simulink model "Modele_Lineaire_Asservi"  (R2024a)
settings: Solver=VariableStepAuto  StartTime=0.0  StopTime=10  RelTol=1e-3
values from neighbouring files (symbols this model uses):
  den_bille_simu = [5*L_plaque 0]    [Code.m]    (also in Initialisation.m = [7*L_plaque 0])
  den_mot_simu = [R_m*J_eq  (R_m*B_eq+n_g*n_m*k_m*k_t*K_g.^2)]    [Code.m]    (also in Initialisation.m)
  Fig_in = 0    [Code.m]
  Frequence = pi    (= 3.14159265359)    [Code.m]
  K_int = real((((-1)*den_mot(1)*(Inter^2)) + ((-1)*den_mot(2)*(Inter^1))) / (num_mot(1)))    [Code.m]    (also in Initialisation.m)
  num_bille_simu = [3*g*r_arm]    [Code.m]    (also in Initialisation.m = [5*g*r_arm])
  num_mot_simu = [K_g*n_m*n_g*k_t]    [Code.m]    (also in Initialisation.m)
  Test_Position = 0.06    [Code.m]    (also in Initialisation.m)
  X_den = TF_PD_Bode_Den    [Code.m]    (also in Initialisation.m)
  X_num = TF_PD_Bode_Num    [Code.m]    (also in Initialisation.m)
settings Model: Creator=francoisdesautels  LastModifiedBy=francoisdesautels

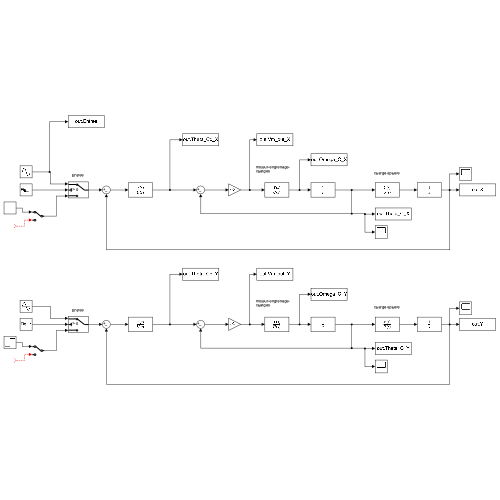
[thumbnail: Simulink's stored preview of the top-level diagram]
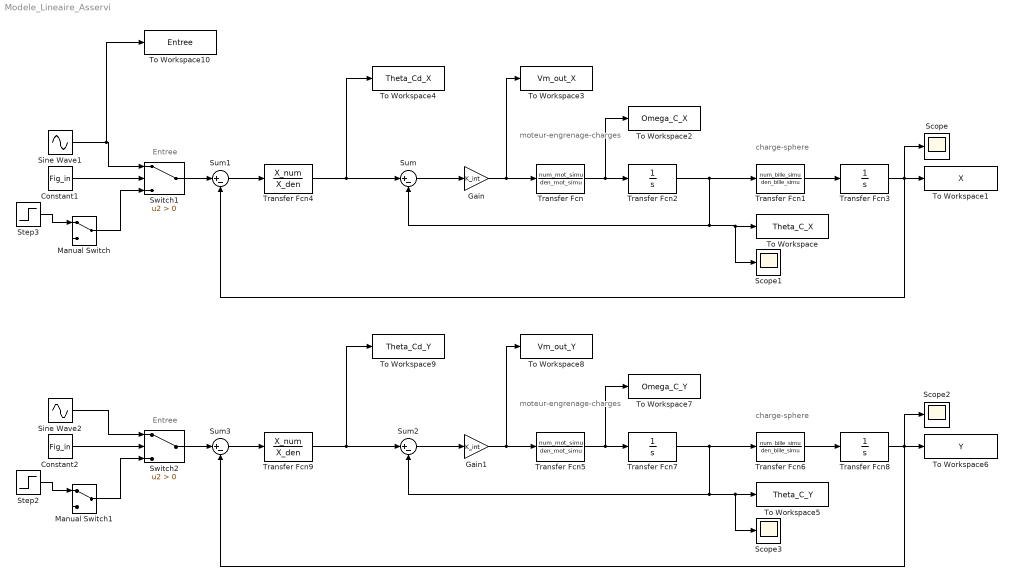
== system Modele_Lineaire_Asservi ==
  note: charge-sphere
  note: moteur-engrenage-charges
  note: moteur-engrenage-charges
  note: charge-sphere
  note: Entree
  note: Entree
  Constant1 : Constant  Value=Fig_in
  Constant2 : Constant  Value=Fig_in
  Gain : Gain  Gain=K_int
  Gain1 : Gain  Gain=K_int
  Manual Switch : ManualSwitch
  Manual Switch1 : ManualSwitch
  Scope{,1..3} (4 alike) : Scope
  Sine Wave1 : Sin  Amplitude=Test_Position  Frequency=Frequence  SampleTime=0
  Sine Wave2 : Sin  Amplitude=Test_Position  Frequency=Frequence  SampleTime=0
  Step2 : Step  After=Test_Position  SampleTime=0
  Step3 : Step  After=Test_Position  SampleTime=0
  Sum{,1..3} (4 alike) : Sum  Inputs=|+-
  Switch1 : Switch  Criteria=u2 > Threshold  SaturateOnIntegerOverflow=off  InputSameDT=off
  Switch2 : Switch  Criteria=u2 > Threshold  SaturateOnIntegerOverflow=off  InputSameDT=off
  To Workspace : ToWorkspace  VariableName=Theta_C_X  SaveFormat=Timeseries  SampleTime=-1
      settings: Save2DSignal=2-D array (concatenate along first dimension)
  To Workspace1 : ToWorkspace  VariableName=X  SaveFormat=Timeseries  SampleTime=-1
  To Workspace10 : ToWorkspace  VariableName=Entree  SaveFormat=Timeseries  SampleTime=-1
      settings: Save2DSignal=2-D array (concatenate along first dimension)
  To Workspace2 : ToWorkspace  VariableName=Omega_C_X  SaveFormat=Timeseries  SampleTime=-1
  To Workspace3 : ToWorkspace  VariableName=Vm_out_X  SaveFormat=Timeseries  SampleTime=-1
      settings: Save2DSignal=2-D array (concatenate along first dimension)
  To Workspace4 : ToWorkspace  VariableName=Theta_Cd_X  SaveFormat=Timeseries  SampleTime=-1
      settings: Save2DSignal=2-D array (concatenate along first dimension)
  To Workspace5 : ToWorkspace  VariableName=Theta_C_Y  SaveFormat=Timeseries  SampleTime=-1
      settings: Save2DSignal=2-D array (concatenate along first dimension)
  To Workspace6 : ToWorkspace  VariableName=Y  SaveFormat=Timeseries  SampleTime=-1
  To Workspace7 : ToWorkspace  VariableName=Omega_C_Y  SaveFormat=Timeseries  SampleTime=-1
  To Workspace8 : ToWorkspace  VariableName=Vm_out_Y  SaveFormat=Timeseries  SampleTime=-1
      settings: Save2DSignal=2-D array (concatenate along first dimension)
  To Workspace9 : ToWorkspace  VariableName=Theta_Cd_Y  SaveFormat=Timeseries  SampleTime=-1
      settings: Save2DSignal=2-D array (concatenate along first dimension)
  Transfer Fcn : TransferFcn  Numerator=num_mot_simu  Denominator=den_mot_simu
  Transfer Fcn1 : TransferFcn  Numerator=num_bille_simu  Denominator=den_bille_simu
  Transfer Fcn{2..3,7..8} (4 alike) : TransferFcn  Denominator=[1 0]
  Transfer Fcn4 : TransferFcn  Numerator=X_num  Denominator=X_den
  Transfer Fcn5 : TransferFcn  Numerator=num_mot_simu  Denominator=den_mot_simu
  Transfer Fcn6 : TransferFcn  Numerator=num_bille_simu  Denominator=den_bille_simu
  Transfer Fcn9 : TransferFcn  Numerator=X_num  Denominator=X_den
  wires:
  Transfer Fcn/1 -> To Workspace2/1, Transfer Fcn2/1
  Transfer Fcn1/1 -> Transfer Fcn3/1
  Transfer Fcn2/1 -> Scope1/1, To Workspace/1, Sum/2, Transfer Fcn1/1
  Transfer Fcn3/1 -> Sum1/2, To Workspace1/1, Scope/1
  Sum/1 -> Gain/1
  Gain/1 -> To Workspace3/1, Transfer Fcn/1
  Transfer Fcn4/1 -> To Workspace4/1, Sum/1
  Sum1/1 -> Transfer Fcn4/1
  Transfer Fcn5/1 -> To Workspace7/1, Transfer Fcn7/1
  Transfer Fcn6/1 -> Transfer Fcn8/1
  Transfer Fcn8/1 -> Sum3/2, To Workspace6/1, Scope2/1
  Sum3/1 -> Transfer Fcn9/1
  Gain1/1 -> To Workspace8/1, Transfer Fcn5/1
  Transfer Fcn7/1 -> Scope3/1, To Workspace5/1, Sum2/2, Transfer Fcn6/1
  Sum2/1 -> Gain1/1
  Transfer Fcn9/1 -> To Workspace9/1, Sum2/1
  Constant1/1 -> Switch1/2
  Sine Wave1/1 -> To Workspace10/1, Switch1/1
  Switch1/1 -> Sum1/1
  Constant2/1 -> Switch2/2
  Sine Wave2/1 -> Switch2/1
  Switch2/1 -> Sum3/1
  Manual Switch/1 -> Switch1/3
  Step3/1 -> Manual Switch/1
  ? -> Manual Switch/2
  Manual Switch1/1 -> Switch2/3
  Step2/1 -> Manual Switch1/1
  ? -> Manual Switch1/2
